simulink model "coupled_tanks_quick_start"  (Simulink 8.3)
settings: Solver=ode1  StartTime=0.0  StopTime=inf  FixedStep=0.1  RelTol=1e-3
PostLoadFcn:
  | qc_set_target_type(getConfigSet(bdroot, 'QUARC Default Target Configuration'));
undefined symbols (not defined in the file or in its folder): HIL
libraries: quarc_library x3
settings Model: Creator=MLevis  LastModifiedBy=Aluno  SimulationMode=external  ExtModeTrigDuration=30000
settings SolverCC: PositivePriorityOrder=on
settings OptimizationCC: ExpressionDepthLimit=2147483647  InitFltsAndDblsToZero=on
settings DebuggingCC: SaveWithParameterizedLinksMsg=none  MultiTaskDSMMsg=warning  MultiTaskCondExecSysMsg=none  FcnCallInpInsideContextMsg=UseLocalSettings
settings RTWCC: SystemTargetFile=quarc_win64.tlc  TemplateMakefile=quarc_default_tmf  Description=QUARC Win64 Target  ProcessScript=quarc_win64_make_rtw_hook
settings STFCustomTargetCC: TargetPreCompLibLocation=C:\PROGRA~3\QUARC\lib\2014a\win64\release  ConcurrentExecutionCompliant=on  GeneratePreprocessorConditionals=Disable all  CPPClassGenCompliant=on  SystemTargetFile=quarc_win64.tlc
settings GRTTargetCC: TargetPreCompLibLocation=C:\PROGRA~3\QUARC\lib\2014a\win64\release  ParMdlRefBuildCompliant=off  CompOptLevelCompliant=off  MatFileLogging=off  ExtMode=on  ExtModeMexFile=quarc_comm

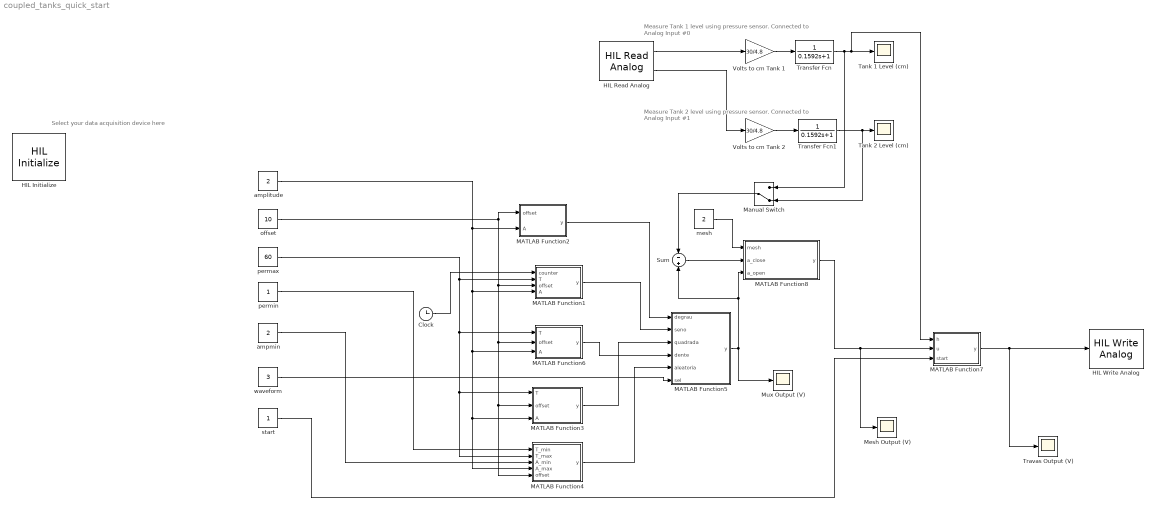
== system coupled_tanks_quick_start ==
  note: Measure Tank 2 level using pressure sensor.
      | Connected to Analog Input #1
  note: Measure Tank 1 level using pressure sensor.
      | Connected to Analog Input #0
  note: Select your data acquisition device here
  Clock : Clock
  HIL Initialize : quarc_library/Data Acquisition/Generic/Configuration/HIL Initialize  object_name=HIL-1  board_type=q2_usb  board_number=0  board_options=d0=digital;d1=digital;led=auto;update_rate=normal;decimation=1  exclusive=off  active=off  hardware_clocks=[0]  clock_modes=[]  initial_clock_frequencies=[]  set_clock_params_at_start=off  set_clock_params_at_switch_in=off  set_clock_frequencies_at_start=off  set_clock_frequencies_at_switch_in=off  analog_input_channels=[0:1]  analog_input_maximums=10  analog_input_minimums=-10  set_analog_input_params_at_start=on  set_analog_input_params_at_switch_in=off  analog_output_channels=[0:1]  analog_output_maximums=10  analog_output_minimums=-10  initial_analog_outputs=[0]  final_analog_outputs=[0]  watchdog_analog_outputs=0  set_analog_output_params_at_start=on  set_analog_output_params_at_switch_in=off  set_analog_outputs_at_start=on  set_analog_outputs_at_switch_in=off  set_analog_outputs_at_terminate=on  set_analog_outputs_at_switch_out=off  set_analog_outputs_on_watchdog=off  digital_input_channels=[]  digital_output_channels=[]  digital_output_configuration=[]  initial_digital_outputs=[1]  final_digital_outputs=[1]  watchdog_digital_outputs=[1]  set_digital_output_params_at_start=off  set_digital_output_params_at_switch_in=off  set_digital_outputs_at_start=on  set_digital_outputs_at_switch_in=off  set_digital_outputs_at_terminate=on  set_digital_outputs_at_switch_out=off  set_digital_outputs_on_watchdog=off  encoder_channels=[0:1]  quadrature=[4]  encoder_filter_frequency=[]  initial_encoder_counts=[0]  set_encoder_params_at_start=on  set_encoder_params_at_switch_in=off  set_encoder_counts_at_start=on  set_encoder_counts_at_switch_in=off  pwm_channels=[]  pwm_modes=[0]  pwm_frequency=1/0.020  pwm_configuration=[]  pwm_alignment=[]  pwm_polarity=[]  pwm_leading_deadband=[]  pwm_trailing_deadband=[]  initial_pwm_outputs=[0]  final_pwm_outputs=[0]  watchdog_pwm_outputs=[0]  set_pwm_params_at_start=on  set_pwm_params_at_switch_in=off  set_pwm_outputs_at_start=on  set_pwm_outputs_at_switch_in=off  set_pwm_outputs_at_terminate=on  set_pwm_outputs_at_switch_out=off  set_pwm_outputs_on_watchdog=off  other_output_channels=[]  initial_other_outputs=[]  final_other_outputs=[]  watchdog_other_outputs=[]  set_other_outputs_at_start=off  set_other_outputs_at_switch_in=off  set_other_outputs_at_terminate=off  set_other_outputs_at_switch_out=off  set_other_outputs_on_watchdog=off
  HIL Read Analog : quarc_library/Data Acquisition/Generic/Immediate I//O/HIL Read Analog  object_name=HIL-1  channels=[0:1]  sample_time=qc_get_step_size  active=on  vector_output=off
  HIL Write Analog : quarc_library/Data Acquisition/Generic/Immediate I//O/HIL Write Analog  object_name=HIL-1  channels=0  sample_time=-1  active=off  vector_input=off
  MATLAB Function1 : MATLAB Function  TreatAsAtomicUnit=on
  MATLAB Function2 : MATLAB Function  TreatAsAtomicUnit=on
  MATLAB Function3 : MATLAB Function  TreatAsAtomicUnit=on
  MATLAB Function4 : MATLAB Function  TreatAsAtomicUnit=on
  MATLAB Function5 : MATLAB Function  TreatAsAtomicUnit=on
  MATLAB Function6 : MATLAB Function  TreatAsAtomicUnit=on
  MATLAB Function7 : MATLAB Function  TreatAsAtomicUnit=on
  MATLAB Function8 : MATLAB Function  TreatAsAtomicUnit=on
  Manual Switch : ManualSwitch  CurrentSetting=0
  Mesh Output (V) : Scope
      settings: TimeRange=10  YMin=2.5  YMax=10  SaveName=meshoutput
  Mux Output (V) : Scope
      settings: TimeRange=10  YMin=4.125  YMax=4.5  SaveName=muxoutput
  Sum : Sum  Inputs=-+
  Tank 1 Level (cm) : Scope
      settings: TimeRange=30  YMin=8  YMax=10  SaveName=tank1level
  Tank 2 Level (cm) : Scope
      settings: TimeRange=30  YMin=7  YMax=9.75  SaveName=tank2level
  Transfer Fcn : TransferFcn  Denominator=[0.1592 1]
  Transfer Fcn1 : TransferFcn  Denominator=[0.1592 1]
  Travas Output (V) : Scope
      settings: TimeRange=30  YMin=2.5  YMax=4  SaveName=travaoutput
  "Volts to cm Tank 1 " : Gain  Gain=30/4.8
  Volts to cm Tank 2 : Gain  Gain=30/4.8
  "amplitude " : Constant  Value=2
  ampmin : Constant  Value=2
  mesh : Constant  Value=2
  offset : Constant  Value=10
  permax : Constant  Value=60
  permin : Constant
  start : Constant
  waveform : Constant  Value=3
  wires:
  MATLAB Function2/1(y) -> MATLAB Function5/1(degrau)
  MATLAB Function1/1(y) -> MATLAB Function5/2(seno)
  MATLAB Function6/1(y) -> MATLAB Function5/4(dente)
  MATLAB Function3/1(y) -> MATLAB Function5/3(quadrada)
  MATLAB Function4/1(y) -> MATLAB Function5/5(aleatoria)
  offset/1 -> MATLAB Function2/1(offset), MATLAB Function1/3(offset), MATLAB Function4/5(offset), MATLAB Function3/2(offset), MATLAB Function6/2(offset)
  permax/1 -> MATLAB Function4/2(T_max), MATLAB Function3/1(T), MATLAB Function6/1(T), MATLAB Function1/2(T)
  Transfer Fcn/1 -> Manual Switch/1, MATLAB Function7/1(h), Tank 1 Level (cm)/1
  waveform/1 -> MATLAB Function5/6(sel)
  permin/1 -> MATLAB Function4/1(T_min)
  ampmin/1 -> MATLAB Function4/3(A_min)
  start/1 -> MATLAB Function7/3(start)
  Clock/1 -> MATLAB Function1/1(counter)
  HIL Read Analog/1 -> "Volts to cm Tank 1 "/1
  "Volts to cm Tank 1 "/1 -> Transfer Fcn/1
  Transfer Fcn1/1 -> Tank 2 Level (cm)/1, Manual Switch/2
  Volts to cm Tank 2/1 -> Transfer Fcn1/1
  HIL Read Analog/2 -> Volts to cm Tank 2/1
  "amplitude "/1 -> MATLAB Function1/4(A), MATLAB Function6/3(A), MATLAB Function3/3(A), MATLAB Function4/4(A_max), MATLAB Function2/2(A)
  MATLAB Function7/1(y) -> Travas Output (V)/1, HIL Write Analog/1
  mesh/1 -> MATLAB Function8/1(mesh)
  MATLAB Function5/1(y) -> Mux Output (V)/1, Sum/2, MATLAB Function8/3(a_open)
  MATLAB Function8/1(y) -> Mesh Output (V)/1, MATLAB Function7/2(u)
  Sum/1 -> MATLAB Function8/2(a_close)
  Manual Switch/1 -> Sum/1

== matlab function MATLAB Function1 ==
  data: counter input double; y output double; T input double; offset input double; A input double
function y = seno(counter, T, offset, A)

%counter = cast(counter, 'double');

y = A*sin(counter*2*pi/T) + offset;

== matlab function MATLAB Function2 ==
  data: offset input double; y output double; A input double
function y = degrau(offset, A)



y = A + offset;

== matlab function MATLAB Function6 ==
  data: y output double; T input double; offset input double; A input double
function y = dente(T, offset, A)

persistent counter_d;

if isempty(counter_d)
   counter_d = 0; 
end


y = counter_d*A/(10*T) + offset;

counter_d = counter_d + 1;

if (counter_d > T*10)
   counter_d = 0;
end

== matlab function MATLAB Function3 ==
  data: y output double; T input double; offset input double; A input double
function y = quadrada(T, offset, A)

persistent counter_q;

if isempty(counter_q)
   counter_q = 0; 
end

counter_q = counter_q + 1;

if (counter_q <= 5*T)
    y = offset;
elseif (counter_q > 5*T)
    y = A + offset;
else
    y = .5;
end

if (counter_q >= 10*T)
   counter_q = 0; 
end

== matlab function MATLAB Function4 ==
  data: T_min input double; y output double; T_max input double; A_min input double; A_max input double; offset input double
function y = aleatoria(T_min, T_max, A_min, A_max, offset)

persistent T_now;
persistent A_now;
persistent counter_a;

if isempty(counter_a)
    T_now = T_min + (T_max - T_min)*rand;
    A_now = A_min + (A_max - A_min)*rand + offset;
    counter_a = 0;
end

counter_a = counter_a + 1;

y = A_now;

if (counter_a >= T_now*10)
    T_now = T_min + (T_max - T_min)*rand;
    A_now = A_min + (A_max - A_min)*rand + offset;
    counter_a = 0;
end

== matlab function MATLAB Function5 ==
  data: degrau input double; y output double; seno input double; quadrada input double; dente input double; aleatoria input double; sel input double
function y = mux(degrau, seno, quadrada, dente, aleatoria, sel)

switch sel
    case 1
        y = degrau;
    case 2
        y = seno;
    case 3
        y = quadrada;
    case 4
        y = dente;
    case 5
        y = aleatoria;
    otherwise
        y = 0;
end

== matlab function MATLAB Function7 ==
  data: h input double; u input double; y output double; start input double
    function y = travas(h, u, start)
%#codegen
h_max = 30;

%Trava de tensão
if(u < -4)
    u = -4;
end
if(u > 4)
    u = 4;
end

%Trava pra não sugar ar
if(u < 0 & h < 2)
    u = 0;
end

%Trava de transbordamento
% if(h >= h_max - 1.0 & h < h_max - 0.75)
%    u = 0.95*u;
% elseif(h >= h_max - 0.75 & h < h_max - 0.5)
%     u = 0.93*u;
% elseif(h >= h_max - 0.5 & h < h_max - 0.25)
%     u = 0.91*u;
% elseif(h >= h_max - 0.25 & h < h_max)
%     u = 0.88*u;
% elseif(h >= h_max)
%     u = 0;
% end

%
if h >= (h_max-1)
    u = (h_max - h)*u;
end

%
% persistent goingup
% 
% if isempty(goingup)
%    goingup = 1; 
% end
% 
% if goingup == 1
%    if h >= 29
%       u = 0;
%       goingup = 0;
%    end
% else
%     if h <= 25
%        goingup = 1; 
%     else
%        u = 0; 
%     end
% end
    
y = start*u;

== matlab function MATLAB Function8 ==
  data: mesh input double; a_close input double; y output double; a_open input double
function y = sel_mesh(mesh, a_close, a_open)
%#codegen

if(mesh == 1)
    y = a_open;
else
    y = a_close;
end
